simulink library "FPGA_Open_Speech_Tools"  (R2020b)
settings: Solver=VariableStepAuto  StartTime=0.0  StopTime=10.0  RelTol=1e-3
undefined symbols (not defined in the file or in its folder): a, b, c, tableInit
libraries: hdlsllib x159, simulink x26, $bdroot x3
(part 2 of 4)

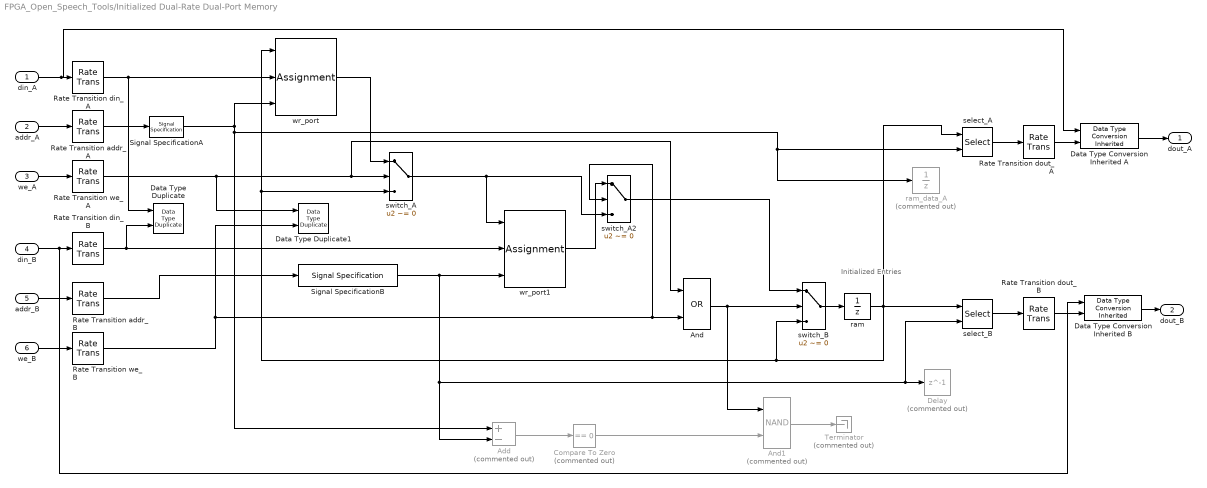
== system FPGA_Open_Speech_Tools/Initialized Dual-Rate Dual-Port Memory ==
  note: Initialized
      | Entries
  din_A : Inport
  addr_A : Inport  Port=2
  we_A : Inport  Port=3  OutDataTypeStr=boolean
  din_B : Inport  Port=4
  addr_B : Inport  Port=5
  we_B : Inport  Port=6  OutDataTypeStr=boolean
  Add : Sum  Commented=on  Inputs=+-
  And : Logic  Operator=OR  AllPortsSameDT=off  OutDataTypeStr=boolean
  And1 : Logic  Commented=on  Operator=NAND  AllPortsSameDT=off  OutDataTypeStr=boolean
  Compare To Zero : simulink/Logic and Bit Operations/Compare To Zero  Commented=on  relop===  OutDataTypeStr=boolean
  Data Type Conversion Inherited A : simulink/Signal Attributes/Data Type Conversion Inherited  ConvertRealWorld=Real World Value  DoSatur=off
      settings: SourceProductBaseCode=SL
  Data Type Conversion Inherited B : simulink/Signal Attributes/Data Type Conversion Inherited  ConvertRealWorld=Real World Value  DoSatur=off
      settings: SourceProductBaseCode=SL
  Data Type Duplicate : DataTypeDuplicate
  Data Type Duplicate1 : DataTypeDuplicate
  Delay : Delay  Commented=on  DelayLength=1
  Rate Transition addr_A : RateTransition  Integrity=off
  Rate Transition addr_B : RateTransition  Integrity=off
  Rate Transition din_A : RateTransition  Integrity=off
  Rate Transition din_B : RateTransition  Integrity=off
  Rate Transition dout_A : RateTransition  Integrity=off
  Rate Transition dout_B : RateTransition  Integrity=off
  Rate Transition we_A : RateTransition  Integrity=off
  Rate Transition we_B : RateTransition  Integrity=off
  Signal SpecificationA : SignalSpecification  OutDataTypeStr=fixdt(0,ram_size,0)  Dimensions=1
  Signal SpecificationB : SignalSpecification  OutDataTypeStr=fixdt(0,ram_size,0)  Dimensions=1
  Terminator : Terminator  Commented=on
      mask Display: disp(sprintf(['Programmable Look-Up Table\nMemory Used: %d bits, Address Width: %d\n' tableFnParam ': %.2d <= x <= %.2d\n Maximum Error: %.2d %%'], 2*2^RAM_SIZE*W_bits, RAM_SIZE, minVal, maxVal, 100*maxErr)); port_label('input',1,'Data_In'); port_label('input',2,'Table_Wr_Data'); port_label('input',3,'Table_RW_Addr'); port_label('input',4,'Table_Wr_En'); port_label('output',1,'Data_Out'); port_label('output',2,'Table_RW_Dout');
  ram : UnitDelay  InitialCondition=Table_Init  SampleTime=-1  HasFrameUpgradeWarning=on
  ram_data_A : UnitDelay  Commented=on  SampleTime=-1  HasFrameUpgradeWarning=on
  select_A : Selector  IndexMode=Zero-based  InputPortWidth=2^ram_size  IndexOptions=Index vector (port)  Indices=[1 3]  OutputSizes=1
  select_B : Selector  IndexMode=Zero-based  InputPortWidth=2^ram_size  IndexOptions=Index vector (port)  Indices=[1 3]  OutputSizes=1
  switch_A : Switch  Criteria=u2 ~= 0
  switch_A2 : Switch  Criteria=u2 ~= 0
  switch_B : Switch  Criteria=u2 ~= 0
  wr_port : Assignment  IndexMode=Zero-based  IndexOptions=Index vector (port)  Indices=1  OutputSizes=[1 1]
  wr_port1 : Assignment  IndexMode=Zero-based  IndexOptions=Index vector (port)  Indices=1  OutputSizes=[1 1]
  dout_A : Outport  VectorParamsAs1DForOutWhenUnconnected=off
  dout_B : Outport  Port=2  VectorParamsAs1DForOutWhenUnconnected=off
  wires:
  Data Type Conversion Inherited A/1 -> dout_A/1
  wr_port1/1 -> switch_A2/1
  Rate Transition dout_A/1 -> Data Type Conversion Inherited A/2
  Data Type Conversion Inherited B/1 -> dout_B/1
  select_B/1 -> Rate Transition dout_B/1
  And/1 -> And1/1, switch_B/2
  Rate Transition addr_A/1 -> Signal SpecificationA/1
  Rate Transition we_A/1 -> And/1, switch_A/2, Data Type Duplicate1/1
  din_A/1 -> Data Type Conversion Inherited A/1, Rate Transition din_A/1
  addr_A/1 -> Rate Transition addr_A/1
  Rate Transition din_B/1 -> wr_port1/2, Data Type Duplicate/2
  switch_A/1 -> wr_port1/1, switch_A2/3
  Signal SpecificationB/1 -> Add/2, select_B/2, Delay/1, wr_port1/3
  switch_A2/1 -> switch_B/1
  Rate Transition din_A/1 -> Data Type Duplicate/1, wr_port/2
  addr_B/1 -> Rate Transition addr_B/1
  switch_B/1 -> ram/1
  Rate Transition dout_B/1 -> Data Type Conversion Inherited B/2
  And1/1 -> Terminator/1
  Add/1 -> Compare To Zero/1
  Compare To Zero/1 -> And1/2
  select_A/1 -> Rate Transition dout_A/1
  ram/1 -> select_B/1, switch_B/3, switch_A/3, wr_port/1, select_A/1
  we_B/1 -> Rate Transition we_B/1
  Signal SpecificationA/1 -> select_A/2, ram_data_A/1, Add/1, wr_port/3
  wr_port/1 -> switch_A/1
  Rate Transition we_B/1 -> switch_A2/2, And/2, Data Type Duplicate1/2
  Rate Transition addr_B/1 -> Signal SpecificationB/1
  din_B/1 -> Data Type Conversion Inherited B/1, Rate Transition din_B/1
  we_A/1 -> Rate Transition we_A/1

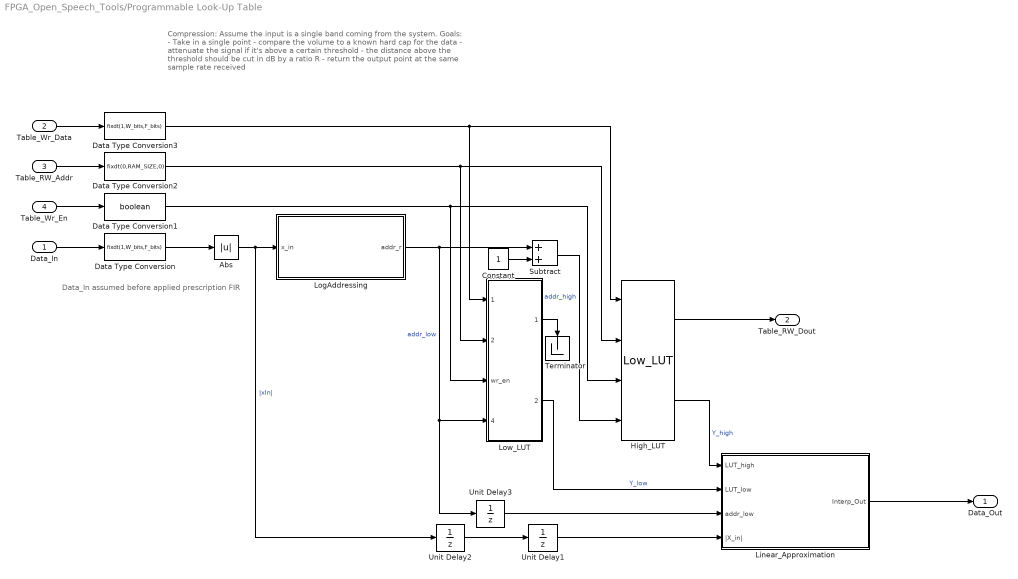
== system FPGA_Open_Speech_Tools/Programmable Look-Up Table ==
  note: Data_In assumed before applied prescription FIR
  note: Compression: Assume the input is a single band coming from the system.
      |
      | Goals:
      | 	- Take in a single point
      | 	- compare the volume to a known hard cap for the data
      | 	- attenuate the signal if it's above a certain threshold
      | 		- the distance above the threshold should be cut in dB by a ratio R
      | 	- return the output point at the same sample rate received
  Data_In : Inport
  Table_Wr_Data : Inport  Port=2
  Table_RW_Addr : Inport  Port=3
  Table_Wr_En : Inport  Port=4
  Abs : Abs
  Constant : Constant  OutDataTypeStr=fixdt(0,RAM_SIZE,0)  SampleTime=-1
  Data Type Conversion : DataTypeConversion  OutDataTypeStr=fixdt(1,W_bits,F_bits)
  Data Type Conversion1 : DataTypeConversion  OutDataTypeStr=boolean
  Data Type Conversion2 : DataTypeConversion  OutDataTypeStr=fixdt(0,RAM_SIZE,0)
  Data Type Conversion3 : DataTypeConversion  OutDataTypeStr=fixdt(1,W_bits,F_bits)
  High_LUT : $bdroot/Programmable Look-Up Table/Low_LUT  ram_size=RAM_SIZE  Table_Init=tableInit
  Linear_Approximation : Subsystem
  LogAddressing : Subsystem
  Low_LUT : Subsystem  mask(Dual-port RAM){ram_size=RAM_SIZE, Table_Init=tableInit}
      mask prompts: ram_size "Address port width (2 to 29 bits)"; Table_Init "Table Initialized Values"
      mask help: This block simulates a dual-port RAM with two data output ports.
      mask init:
      | hdlblkmask_dpram;
      mask Help: helpview([docroot '/simulink/helptargets.map'],'HDL_dual_port_RAM');
  Subtract : Sum  OutDataTypeStr=Inherit: Same as first input
  Terminator : Terminator
  Unit Delay1 : UnitDelay  InitialCondition=1  SampleTime=-1  HasFrameUpgradeWarning=on
  Unit Delay2 : UnitDelay  InitialCondition=1  SampleTime=-1  HasFrameUpgradeWarning=on
  Unit Delay3 : UnitDelay  InitialCondition=1  SampleTime=-1  HasFrameUpgradeWarning=on
  Data_Out : Outport  VectorParamsAs1DForOutWhenUnconnected=off
  Table_RW_Dout : Outport  Port=2  VectorParamsAs1DForOutWhenUnconnected=off
  wires:
  Table_Wr_Data/1 -> Data Type Conversion3/1
  Table_Wr_En/1 -> Data Type Conversion1/1
  Table_RW_Addr/1 -> Data Type Conversion2/1
  LogAddressing/1(addr_r) -> Unit Delay3/1, Low_LUT/4(rd_addr), Subtract/1  "addr_low"
  Abs/1 -> Unit Delay2/1, LogAddressing/1(x_in)  "|xIn|"
  Data_In/1 -> Data Type Conversion/1
  Constant/1 -> Subtract/2
  Subtract/1 -> High_LUT/4  "addr_high"
  Low_LUT/1(wr_dout) -> Terminator/1
  High_LUT/1 -> Table_RW_Dout/1
  High_LUT/2 -> Linear_Approximation/1(LUT_high)  "Y_high"
  Low_LUT/2(rd_dout) -> Linear_Approximation/2(LUT_low)  "Y_low"
  Linear_Approximation/1(Interp_Out) -> Data_Out/1
  Unit Delay2/1 -> Unit Delay1/1
  Unit Delay1/1 -> Linear_Approximation/4(|X_in|)
  Unit Delay3/1 -> Linear_Approximation/3(addr_low)
  Data Type Conversion/1 -> Abs/1
  Data Type Conversion1/1 -> High_LUT/3, Low_LUT/3(wr_en)
  Data Type Conversion2/1 -> High_LUT/2, Low_LUT/2(wr_addr)
  Data Type Conversion3/1 -> High_LUT/1, Low_LUT/1(wr_din)

== system FPGA_Open_Speech_Tools/Programmable Look-Up Table, Linear Scale ==
  note: Data_In assumed before applied prescription FIR
  note: Compression: Assume the input is a single band coming from the system.
      |
      | Goals:
      | 	- Take in a single point
      | 	- compare the volume to a known hard cap for the data
      | 	- attenuate the signal if it's above a certain threshold
      | 		- the distance above the threshold should be cut in dB by a ratio R
      | 	- return the output point at the same sample rate received
  Data_In : Inport
  Table_Wr_Data : Inport  Port=2
  Table_Wr_Addr : Inport  Port=3
  Table_Wr_En : Inport  Port=4
  Data Type Conversion : DataTypeConversion  OutDataTypeStr=fixdt(isSigned,W_bits,F_bits)
  Data Type Conversion1 : DataTypeConversion  OutDataTypeStr=boolean
  Data Type Conversion2 : DataTypeConversion  OutDataTypeStr=fixdt(0,RAM_SIZE,0)
  Data Type Conversion3 : DataTypeConversion  OutDataTypeStr=fixdt(1,W_bits,F_bits)
  LinAddressing : Subsystem
  Low_LUT : Subsystem  mask(Dual-port RAM){ram_size=RAM_SIZE, Table_Init=tableInit}
      mask prompts: ram_size "Address port width (2 to 29 bits)"; Table_Init "Table Initialized Values"
      mask help: This block simulates a dual-port RAM with two data output ports.
      mask init:
      | hdlblkmask_dpram;
      mask Help: helpview([docroot '/simulink/helptargets.map'],'HDL_dual_port_RAM');
  Data_Out : Outport  VectorParamsAs1DForOutWhenUnconnected=off
  Table_RW_Dout : Outport  Port=2  VectorParamsAs1DForOutWhenUnconnected=off
  wires:
  Table_Wr_Data/1 -> Data Type Conversion3/1
  Table_Wr_En/1 -> Data Type Conversion1/1
  Table_Wr_Addr/1 -> Data Type Conversion2/1
  LinAddressing/1(addr_r) -> Low_LUT/4(rd_addr)  "addr"
  Data Type Conversion/1 -> LinAddressing/1(x_in)  "x_in"
  Data_In/1 -> Data Type Conversion/1
  Low_LUT/1(wr_dout) -> Table_RW_Dout/1
  Data Type Conversion1/1 -> Low_LUT/3(wr_en)
  Data Type Conversion2/1 -> Low_LUT/2(wr_addr)
  Data Type Conversion3/1 -> Low_LUT/1(wr_din)
  Low_LUT/2(rd_dout) -> Data_Out/1  "Y_low"

== system FPGA_Open_Speech_Tools/Programmable Lookup Table dB ==
  note: Data_In assumed before applied prescription FIR
  note: Compression: Assume the input is a single band coming from the system.
      |
      | Goals:
      | 	- Take in a single point
      | 	- compare the volume to a known hard cap for the data
      | 	- attenuate the signal if it's above a certain threshold
      | 		- the distance above the threshold should be cut in dB by a ratio R
      | 	- return the output point at the same sample rate received
  Data_In : Inport
  Table_Wr_Data : Inport  Port=2
  Table_RW_Addr : Inport  Port=3
  Table_Wr_En : Inport  Port=4
  Abs : Abs
  Constant : Constant  OutDataTypeStr=fixdt(0,RAM_SIZE,0)  SampleTime=-1
  Data Type Conversion : DataTypeConversion  OutDataTypeStr=fixdt(1,W_bits,F_bits)
  Data Type Conversion1 : DataTypeConversion  OutDataTypeStr=boolean
  Data Type Conversion2 : DataTypeConversion  OutDataTypeStr=fixdt(0,RAM_SIZE,0)
  Data Type Conversion3 : DataTypeConversion  OutDataTypeStr=fixdt(1,W_bits,F_bits-5)
  High_LUT : $bdroot/Programmable Look-Up Table/Low_LUT  ram_size=RAM_SIZE  Table_Init=tableInit
  Linear_Approximation : Subsystem  AncestorBlock=FPGA_Open_Speech_Tools/Programmable Look-Up Table/Linear_Approximation
  LogAddressing : Subsystem  AncestorBlock=FPGA_Open_Speech_Tools/Programmable Look-Up Table/LogAddressing
  Low_LUT : $bdroot/Programmable Look-Up Table/Low_LUT  ram_size=RAM_SIZE  Table_Init=tableInit
  Subtract : Sum  OutDataTypeStr=Inherit: Same as first input
  Terminator : Terminator
  Unit Delay1 : UnitDelay  InitialCondition=1  SampleTime=-1  HasFrameUpgradeWarning=on
  Unit Delay2 : UnitDelay  InitialCondition=1  SampleTime=-1  HasFrameUpgradeWarning=on
  Unit Delay3 : UnitDelay  InitialCondition=1  SampleTime=-1  HasFrameUpgradeWarning=on
  Data_Out : Outport  VectorParamsAs1DForOutWhenUnconnected=off
  Table_RW_Dout : Outport  Port=2  VectorParamsAs1DForOutWhenUnconnected=off
  wires:
  Data Type Conversion1/1 -> High_LUT/3, Low_LUT/3
  Table_RW_Addr/1 -> Data Type Conversion2/1
  Data Type Conversion3/1 -> High_LUT/1, Low_LUT/1
  Constant/1 -> Subtract/2
  Table_Wr_En/1 -> Data Type Conversion1/1
  High_LUT/2 -> Linear_Approximation/1(LUT_high)  "Y_high"
  LogAddressing/1(addr_r) -> Unit Delay3/1, Low_LUT/4, Subtract/1  "addr_low"
  High_LUT/1 -> Table_RW_Dout/1
  Subtract/1 -> High_LUT/4  "addr_high"
  Data Type Conversion/1 -> Abs/1
  Unit Delay1/1 -> Linear_Approximation/4(|X_in|)
  Low_LUT/1 -> Terminator/1
  Low_LUT/2 -> Linear_Approximation/2(LUT_low)  "Y_low"
  Unit Delay3/1 -> Linear_Approximation/3(addr_low)
  Abs/1 -> Unit Delay2/1, LogAddressing/1(x_in)  "|xIn|"
  Data Type Conversion2/1 -> High_LUT/2, Low_LUT/2
  Linear_Approximation/1(Interp_Out) -> Data_Out/1
  Unit Delay2/1 -> Unit Delay1/1
  Data_In/1 -> Data Type Conversion/1
  Table_Wr_Data/1 -> Data Type Conversion3/1

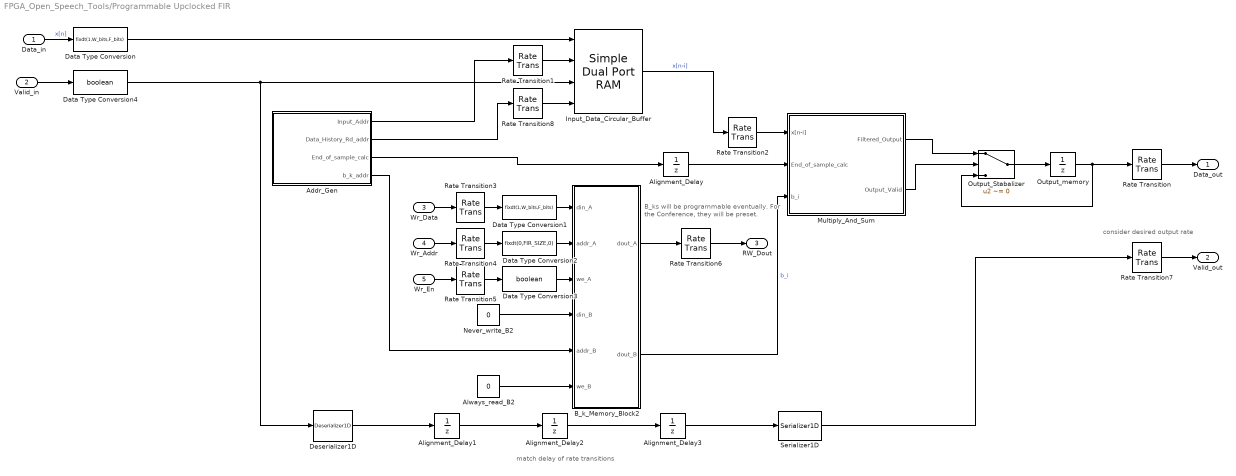
== system FPGA_Open_Speech_Tools/Programmable Upclocked FIR ==
  note: match delay of rate transitions
  note: consider desired output rate
  note: B_ks will be programmable eventually.
      | For the Conference, they will be preset.
  Data_in : Inport
  Valid_in : Inport  Port=2
  Wr_Data : Inport  Port=3
  Wr_Addr : Inport  Port=4
  Wr_En : Inport  Port=5
  "Addr_Gen " : Subsystem
  Alignment_Delay{,1..3} (4 alike) : UnitDelay  SampleTime=-1  HasFrameUpgradeWarning=on
  Always_read_B2 : Constant  Value=0  OutDataTypeStr=boolean  SampleTime=Ts/FIR_UPRATE
  B_k_Memory_Block2 : Subsystem  mask(Dual-rate dual-port RAM){ram_size=FIR_SIZE, B_k_init=firCoeff}
      mask prompts: ram_size "Address port width (2 to 28 bits)"
      mask help: This block simulates a dual-clock dual-port RAM with two data output ports.
      mask init:
      | hdlblkmask_drdpram();
      mask Help: helpview([docroot '/simulink/helptargets.map'],'HDL_dual_rate_dual_port_ram');
  Data Type Conversion : DataTypeConversion  OutDataTypeStr=fixdt(1,W_bits,F_bits)
  Data Type Conversion1 : DataTypeConversion  OutDataTypeStr=fixdt(1,W_bits,F_bits)
  Data Type Conversion2 : DataTypeConversion  OutDataTypeStr=fixdt(0,FIR_SIZE,0)
  Data Type Conversion3 : DataTypeConversion  OutDataTypeStr=boolean
  Data Type Conversion4 : DataTypeConversion  OutDataTypeStr=boolean
  Deserializer1D : hdlsllib/HDL Operations/Deserializer1D  Ratio=(1/maxRate)/Ts_system  IdleCycles=0  InitialCondition=0  startIn=off  validIn=off  validOut=off  inputDataDimensions=-1  inputSampleTime=-1  inputSignalType=auto
      settings: SourceProductBaseCode=SL
  Input_Data_Circular_Buffer : hdlsllib/HDL RAMs/Simple Dual Port RAM  ram_size=FIR_SIZE
      settings: SourceProductBaseCode=SL
  Multiply_And_Sum : Subsystem
  Never_write_B2 : Constant  Value=0  OutDataTypeStr=fixdt(1, W_bits, F_bits)  SampleTime=Ts/FIR_UPRATE
  Output_Stabalizer : Switch  Criteria=u2 ~= 0
  Output_memory : UnitDelay  SampleTime=-1  HasFrameUpgradeWarning=on
  Rate Transition{,1,6..8} (5 alike) : RateTransition  OutPortSampleTime=Ts_system
  Rate Transition{2..5} (4 alike) : RateTransition  OutPortSampleTime=Ts/FIR_UPRATE
  Serializer1D : hdlsllib/HDL Operations/Serializer1D  Ratio=(1/maxRate)/Ts_system  IdleCycles=0  validIn=off  startOut=off  validOut=off  inputDataDimensions=-1  inputSampleTime=-1  inputSignalType=auto
      settings: SourceProductBaseCode=SL
  Data_out : Outport  VectorParamsAs1DForOutWhenUnconnected=off
  Valid_out : Outport  Port=2  VectorParamsAs1DForOutWhenUnconnected=off
  RW_Dout : Outport  Port=3  VectorParamsAs1DForOutWhenUnconnected=off
  wires:
  Alignment_Delay/1 -> Multiply_And_Sum/2(End_of_sample_calc)
  "Addr_Gen "/4(b_k_addr) -> B_k_Memory_Block2/5(addr_B)
  Output_memory/1 -> Rate Transition/1, Output_Stabalizer/3
  Valid_in/1 -> Data Type Conversion4/1
  Never_write_B2/1 -> B_k_Memory_Block2/4(din_B)
  Multiply_And_Sum/1(Filtered_Output) -> Output_Stabalizer/1
  Data_in/1 -> Data Type Conversion/1  "x[n]"
  "Addr_Gen "/3(End_of_sample_calc) -> Alignment_Delay/1
  B_k_Memory_Block2/2(dout_B) -> Multiply_And_Sum/3(b_i)  "b_i"
  "Addr_Gen "/1(Input_Addr) -> Rate Transition1/1
  Output_Stabalizer/1 -> Output_memory/1
  "Addr_Gen "/2(Data_History_Rd_addr) -> Rate Transition8/1
  Rate Transition4/1 -> Data Type Conversion2/1
  Input_Data_Circular_Buffer/1 -> Rate Transition2/1  "x[n-i]"
  Rate Transition3/1 -> Data Type Conversion1/1
  Always_read_B2/1 -> B_k_Memory_Block2/6(we_B)
  Rate Transition/1 -> Data_out/1
  Wr_Data/1 -> Rate Transition3/1
  Wr_Addr/1 -> Rate Transition4/1
  Rate Transition5/1 -> Data Type Conversion3/1
  Wr_En/1 -> Rate Transition5/1
  B_k_Memory_Block2/1(dout_A) -> Rate Transition6/1
  Rate Transition6/1 -> RW_Dout/1
  Rate Transition7/1 -> Valid_out/1
  Data Type Conversion1/1 -> B_k_Memory_Block2/1(din_A)
  Data Type Conversion2/1 -> B_k_Memory_Block2/2(addr_A)
  Data Type Conversion3/1 -> B_k_Memory_Block2/3(we_A)
  Multiply_And_Sum/2(Output_Valid) -> Output_Stabalizer/2
  Data Type Conversion4/1 -> Deserializer1D/1, Input_Data_Circular_Buffer/3
  Data Type Conversion/1 -> Input_Data_Circular_Buffer/1
  Deserializer1D/1 -> Alignment_Delay1/1
  Serializer1D/1 -> Rate Transition7/1
  Rate Transition2/1 -> Multiply_And_Sum/1(x[n-i])
  Rate Transition1/1 -> Input_Data_Circular_Buffer/2
  Rate Transition8/1 -> Input_Data_Circular_Buffer/4
  Alignment_Delay1/1 -> Alignment_Delay2/1
  Alignment_Delay2/1 -> Alignment_Delay3/1
  Alignment_Delay3/1 -> Serializer1D/1

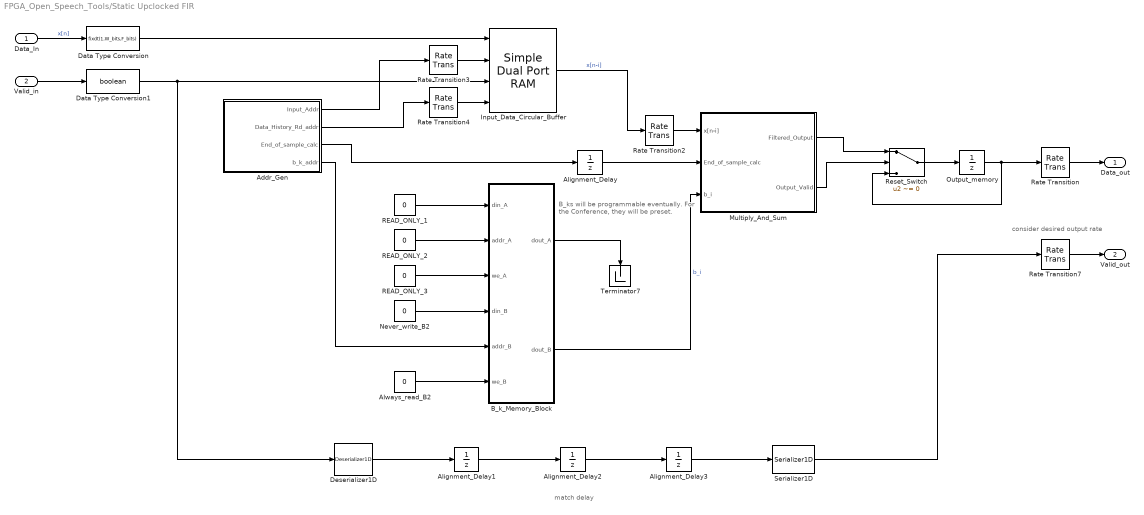
== system FPGA_Open_Speech_Tools/Static Upclocked FIR ==
  note: consider desired output rate
  note: B_ks will be programmable eventually.
      | For the Conference, they will be preset.
  note: match delay
  Data_In : Inport
  Valid_in : Inport  Port=2
  "Addr_Gen " : Subsystem
  Alignment_Delay{,1..3} (4 alike) : UnitDelay  SampleTime=-1  HasFrameUpgradeWarning=on
  Always_read_B2 : Constant  Value=0  OutDataTypeStr=boolean  SampleTime=Ts/FIR_UPRATE
  B_k_Memory_Block : Subsystem  mask(Dual-rate dual-port RAM){ram_size=FIR_SIZE, B_k_init=firCoeff}
      mask prompts: ram_size "Address port width (2 to 28 bits)"
      mask help: This block simulates a dual-clock dual-port RAM with two data output ports.
      mask init:
      | hdlblkmask_drdpram();
      mask Help: helpview([docroot '/simulink/helptargets.map'],'HDL_dual_rate_dual_port_ram');
  Data Type Conversion : DataTypeConversion  OutDataTypeStr=fixdt(1,W_bits,F_bits)
  Data Type Conversion1 : DataTypeConversion  OutDataTypeStr=boolean
  Deserializer1D : hdlsllib/HDL Operations/Deserializer1D  Ratio=(1/maxRate)/Ts_system  IdleCycles=0  InitialCondition=0  startIn=off  validIn=off  validOut=off  inputDataDimensions=-1  inputSampleTime=-1  inputSignalType=auto
      settings: SourceProductBaseCode=SL
  Input_Data_Circular_Buffer : hdlsllib/HDL RAMs/Simple Dual Port RAM  ram_size=FIR_SIZE
      settings: SourceProductBaseCode=SL
  Multiply_And_Sum : Subsystem
  Never_write_B2 : Constant  Value=0  OutDataTypeStr=fixdt(1, W_bits, F_bits)  SampleTime=Ts/FIR_UPRATE
  Output_memory : UnitDelay  SampleTime=-1  HasFrameUpgradeWarning=on
  READ_ONLY_1 : Constant  Value=0  OutDataTypeStr=fixdt(1, W_bits, F_bits)  SampleTime=Ts/FIR_UPRATE
  READ_ONLY_2 : Constant  Value=0  OutDataTypeStr=fixdt(0,FIR_SIZE, 0)  SampleTime=Ts/FIR_UPRATE
  READ_ONLY_3 : Constant  Value=0  OutDataTypeStr=boolean  SampleTime=Ts/FIR_UPRATE
  Rate Transition : RateTransition  OutPortSampleTime=Ts_system
  Rate Transition2 : RateTransition  OutPortSampleTime=Ts/FIR_UPRATE
  Rate Transition3 : RateTransition  OutPortSampleTime=Ts/FIR_UPRATE
  Rate Transition4 : RateTransition  OutPortSampleTime=Ts/FIR_UPRATE
  Rate Transition7 : RateTransition  OutPortSampleTime=Ts_system
  Reset_Switch : Switch  Criteria=u2 ~= 0
  Serializer1D : hdlsllib/HDL Operations/Serializer1D  Ratio=(1/maxRate)/Ts_system  IdleCycles=0  validIn=off  startOut=off  validOut=off  inputDataDimensions=-1  inputSampleTime=-1  inputSignalType=auto
      settings: SourceProductBaseCode=SL
  Terminator7 : Terminator
  Data_out : Outport  VectorParamsAs1DForOutWhenUnconnected=off
  Valid_out : Outport  Port=2  VectorParamsAs1DForOutWhenUnconnected=off
  wires:
  Valid_in/1 -> Data Type Conversion1/1
  Alignment_Delay/1 -> Multiply_And_Sum/2(End_of_sample_calc)
  "Addr_Gen "/4(b_k_addr) -> B_k_Memory_Block/5(addr_B)
  Output_memory/1 -> Rate Transition/1, Reset_Switch/3
  Never_write_B2/1 -> B_k_Memory_Block/4(din_B)
  READ_ONLY_3/1 -> B_k_Memory_Block/3(we_A)
  Multiply_And_Sum/1(Filtered_Output) -> Reset_Switch/1
  Data_In/1 -> Data Type Conversion/1  "x[n]"
  "Addr_Gen "/3(End_of_sample_calc) -> Alignment_Delay/1
  B_k_Memory_Block/2(dout_B) -> Multiply_And_Sum/3(b_i)  "b_i"
  "Addr_Gen "/1(Input_Addr) -> Rate Transition3/1
  Reset_Switch/1 -> Output_memory/1
  "Addr_Gen "/2(Data_History_Rd_addr) -> Rate Transition4/1
  READ_ONLY_2/1 -> B_k_Memory_Block/2(addr_A)
  Input_Data_Circular_Buffer/1 -> Rate Transition2/1  "x[n-i]"
  READ_ONLY_1/1 -> B_k_Memory_Block/1(din_A)
  Multiply_And_Sum/2(Output_Valid) -> Reset_Switch/2
  B_k_Memory_Block/1(dout_A) -> Terminator7/1
  Always_read_B2/1 -> B_k_Memory_Block/6(we_B)
  Rate Transition/1 -> Data_out/1
  Rate Transition7/1 -> Valid_out/1
  Data Type Conversion/1 -> Input_Data_Circular_Buffer/1
  Data Type Conversion1/1 -> Deserializer1D/1, Input_Data_Circular_Buffer/3
  Rate Transition3/1 -> Input_Data_Circular_Buffer/2
  Rate Transition4/1 -> Input_Data_Circular_Buffer/4
  Rate Transition2/1 -> Multiply_And_Sum/1(x[n-i])
  Alignment_Delay2/1 -> Alignment_Delay3/1
  Alignment_Delay3/1 -> Serializer1D/1
  Alignment_Delay1/1 -> Alignment_Delay2/1
  Deserializer1D/1 -> Alignment_Delay1/1
  Serializer1D/1 -> Rate Transition7/1

== system FPGA_Open_Speech_Tools/Variable Delay Block ==
  note: Special Case for Delay = 2^N:
      | If Valid is asserted, we have 1 clock cycle before overwriting the circ buffer data for 2^N samples ago.
      | Readout of circ buffer will be correct for 1 cycle.
      |
      | If valid is not asserted?
      | This means the data for 2^N samples ago has already been overwritten. It's already too late to get that sample.
  note: Solution: Implement Special Case switches to allow for read-first enabled circular buffer 1 cycle to write.
      | Then, use a switch to allow the circ buffer to take back over, preventing non-valid signals from showing on output.
  note: max delay: (2^N) -1
  note: circ buffer is read-first, requiring a switch for delays of 0 and 1
  note: problem: no delay of 1 available with circular buffer
  Data_In : Inport
  Data_Valid : Inport  Port=2
  Delay : Inport  Port=3
  "Addr_Gen " : Subsystem
  Data Type Conversion : DataTypeConversion  OutDataTypeStr=fixdt(0, RAM_SIZE, 0)
  Data Type Conversion1 : DataTypeConversion  OutDataTypeStr=boolean
  Input_Data_Circular_Buffer : Subsystem
  Multiport Switch : MultiPortSwitch  DataPortOrder=Zero-based contiguous  Inputs=2  DataPortIndices={0,2^RAMSIZE}  DiagnosticForDefault=None  zeroidx=on
  Output_Stabalizer_Z0 : Switch  Criteria=u2 ~= 0
  Subtract : Sum  Inputs=+-  OutDataTypeStr=Inherit: Same as first input
  Data_out : Outport  VectorParamsAs1DForOutWhenUnconnected=off
  wires:
  Subtract/1 -> Input_Data_Circular_Buffer/4(rd_addr)
  Data_Valid/1 -> Data Type Conversion1/1
  Input_Data_Circular_Buffer/1(rd_dout) -> Multiport Switch/3, Output_Stabalizer_Z0/3  "x[n-i]"
  Delay/1 -> Data Type Conversion/1
  Multiport Switch/1 -> Data_out/1
  Data Type Conversion/1 -> Multiport Switch/1, Subtract/2
  Data_In/1 -> Input_Data_Circular_Buffer/1(wr_din), Output_Stabalizer_Z0/1
  Data Type Conversion1/1 -> Input_Data_Circular_Buffer/3(wr_en), Output_Stabalizer_Z0/2, "Addr_Gen "/Enable
  Output_Stabalizer_Z0/1 -> Multiport Switch/2
  "Addr_Gen "/1(Input_Addr) -> Subtract/1, Input_Data_Circular_Buffer/2(wr_addr)

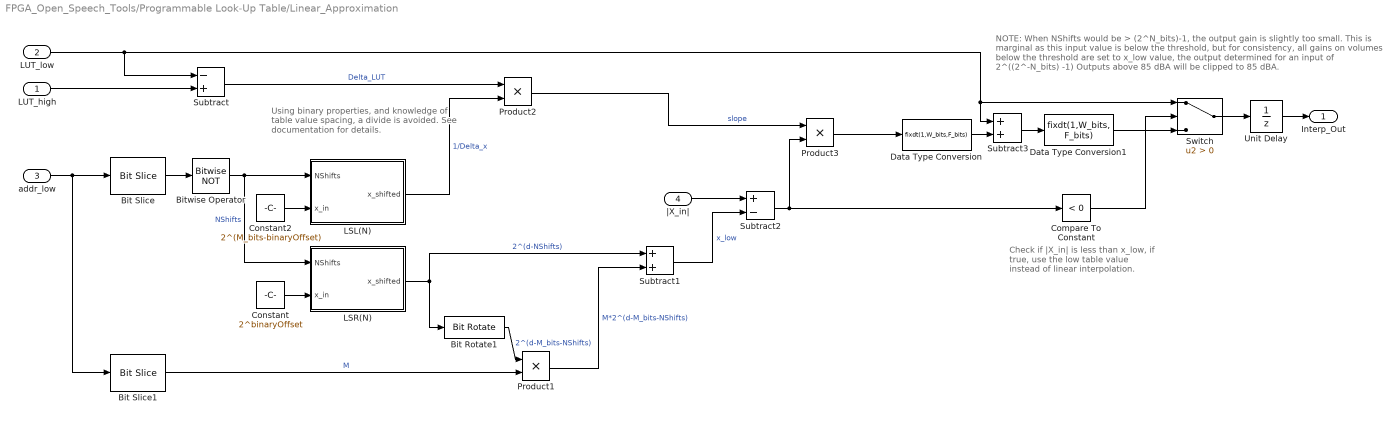
== system FPGA_Open_Speech_Tools/Programmable Look-Up Table/Linear_Approximation ==
  note: Using binary properties, and knowledge
      | of table value spacing, a divide is avoided.
      | See documentation for details.
  note: Check if |X_in| is less than x_low,
      | if true, use the low table value
      | instead of linear interpolation.
  note: NOTE: When NShifts would be > (2^N_bits)-1, the output gain is slightly too small.
      | This is marginal as this input value is below the threshold, but for consistency,
      | all gains on volumes below the threshold are set to x_low value, the output determined
      | for an input of 2^((2^-N_bits)  -1)
      | Outputs above 85 dBA will be clipped to 85 dBA.
  LUT_high : Inport
  LUT_low : Inport  Port=2
  addr_low : Inport  Port=3
  |X_in| : Inport  Port=4
  Bit Rotate1 : hdlsllib/Logic and Bit Operations/Bit Rotate  mode=Rotate Right  N=M_bits
      settings: SourceProductBaseCode=SL
  Bit Slice : hdlsllib/Logic and Bit Operations/Bit Slice  lidx=M_bits+N_bits-1  ridx=M_bits
      settings: SourceProductBaseCode=SL
  Bit Slice1 : hdlsllib/Logic and Bit Operations/Bit Slice  lidx=M_bits-1  ridx=0
      settings: SourceProductBaseCode=SL
  Bitwise Operator : simulink/Logic and Bit Operations/Bitwise Operator  logicop=NOT  UseBitMask=off  BitMask=bin2dec('11011001')  BitMaskRealWorld=Stored Integer
  Compare To Constant : simulink/Logic and Bit Operations/Compare To Constant  relop=<  const=0  OutDataTypeStr=boolean
  Constant : Constant  Value=2^binaryOffset  OutDataTypeStr=fixdt(0,W_bits,W_bits-2)  SampleTime=-1
  Constant2 : Constant  Value=2^(M_bits-binaryOffset)  OutDataTypeStr=fixdt(0,W_bits,0)  SampleTime=-1
  Data Type Conversion : DataTypeConversion  OutDataTypeStr=fixdt(1,W_bits,F_bits)
  Data Type Conversion1 : DataTypeConversion  OutDataTypeStr=fixdt(1,W_bits, F_bits)
  LSL(N) : Subsystem
  LSR(N) : Subsystem
  Product1 : Product
  Product2 : Product
  Product3 : Product
  Subtract : Sum  Inputs=-+  OutDataTypeStr=Inherit: Same as first input
  Subtract1 : Sum  OutDataTypeStr=fixdt(1,W_bits, F_bits)
  Subtract2 : Sum  Inputs=+-  OutDataTypeStr=Inherit: Same as first input
  Subtract3 : Sum
  Switch : Switch  Criteria=u2 > Threshold
  Unit Delay : UnitDelay  InitialCondition=1  SampleTime=-1  HasFrameUpgradeWarning=on
  Interp_Out : Outport  VectorParamsAs1DForOutWhenUnconnected=off
  wires:
  addr_low/1 -> Bit Slice1/1, Bit Slice/1
  Bit Slice/1 -> Bitwise Operator/1
  Bitwise Operator/1 -> LSR(N)/1(NShifts), LSL(N)/1(NShifts)  "NShifts"
  Bit Slice1/1 -> Product1/2  "M"
  LUT_high/1 -> Subtract/2
  LUT_low/1 -> Subtract/1, Switch/1, Subtract3/1
  Subtract/1 -> Product2/1  "Delta_LUT"
  Constant/1 -> LSR(N)/2(x_in)
  LSR(N)/1(x_shifted) -> Subtract1/1, Bit Rotate1/1  "2^(d-NShifts)"
  Bit Rotate1/1 -> Product1/1  "2^(d-M_bits-NShifts)"
  Product1/1 -> Subtract1/2  "M*2^(d-M_bits-NShifts)"
  Subtract1/1 -> Subtract2/2  "x_low"
  LSL(N)/1(x_shifted) -> Product2/2  "1/Delta_x"
  Product2/1 -> Product3/1  "slope"
  |X_in|/1 -> Subtract2/1
  Subtract2/1 -> Compare To Constant/1, Product3/2
  Product3/1 -> Data Type Conversion/1
  Subtract3/1 -> Data Type Conversion1/1
  Constant2/1 -> LSL(N)/2(x_in)
  Data Type Conversion/1 -> Subtract3/2
  Data Type Conversion1/1 -> Switch/3
  Unit Delay/1 -> Interp_Out/1
  Compare To Constant/1 -> Switch/2
  Switch/1 -> Unit Delay/1

== system FPGA_Open_Speech_Tools/Programmable Look-Up Table/LogAddressing ==
  note: z-1 here
      |    	|
      |    	|
      |   	v
  note: If input > highest expected input,
  note: If input < floor threshold input,
      | use the output corresponding to
      | the floor threshold input.
  note: Note: simulation version of this block has no latency.
      | But, in VHDL the inputs are registered, delaying the signal by 1.
      | If testing a simulation, simply attach a unit delay block after the
      | addition and before the signal split.
  note: Have to change size to 40 because
      |  LZC made for 40 bit number
  note: EFFECTIVELY shift_left(x_in,NShifts)
  x_in : Inport
  Bit Concat : hdlsllib/Logic and Bit Operations/Bit Concat  numInputs=2
  Bit Slice : hdlsllib/Logic and Bit Operations/Bit Slice  lidx=N_bits-1  ridx=0
      settings: SourceProductBaseCode=SL
  Bit Slice1 : hdlsllib/Logic and Bit Operations/Bit Slice  lidx=F_bits-1+binaryOffset  ridx=F_bits-M_bits+binaryOffset
      settings: SourceProductBaseCode=SL
  Bitwise Operator1 : simulink/Logic and Bit Operations/Bitwise Operator  logicop=NOT  UseBitMask=off  BitMask=bin2dec('11011001')  BitMaskRealWorld=Stored Integer
  Constant6 : Constant  Value=0  OutDataTypeStr=fixdt(0,RAM_SIZE,0)  SampleTime=-1
  Data Type Conversion : DataTypeConversion  OutDataTypeStr=fixdt(0,40,F_bits+40-W_bits)
  Delay1 : Delay  DelayLength=1  InitialCondition=minVal
  Delay2 : Delay  DelayLength=1  InitialCondition=minVal
  LSL(N) : Subsystem
  MATLAB Function : MATLAB Function  TreatAsAtomicUnit=on
  Offset : Constant  Value=W_bits-1-F_bits-binaryOffset  OutDataTypeStr=fixdt(0,6,0)  SampleTime=-1
  Remove Sign : DataTypeConversion  OutDataTypeStr=fixdt(0,W_bits,F_bits)
  Subtract : Sum  Inputs=+-  OutDataTypeStr=Inherit: Same as first input
  Switch1 : Switch  Criteria=u2 ~= 0
  Threshold Check : simulink/Logic and Bit Operations/Compare To Constant  relop=>  const=2^N_bits -1  OutDataTypeStr=boolean
  addr_r : Outport  VectorParamsAs1DForOutWhenUnconnected=off
  wires:
  x_in/1 -> Remove Sign/1, Data Type Conversion/1
  Bit Slice1/1 -> Bit Concat/2  "M"
  Bitwise Operator1/1 -> Bit Concat/1  "addr(5 downto 2)"
  MATLAB Function/1(lzc_count) -> Subtract/1
  Bit Concat/1 -> Switch1/3
  Offset/1 -> Subtract/2
  Bit Slice/1 -> Bitwise Operator1/1, LSL(N)/1(NShifts)  "NShifts"
  Delay2/1 -> LSL(N)/2(x_in)
  LSL(N)/1(x_shifted) -> Bit Slice1/1
  Data Type Conversion/1 -> MATLAB Function/1(x)
  Constant6/1 -> Switch1/1
  Switch1/1 -> addr_r/1
  Threshold Check/1 -> Switch1/2
  Remove Sign/1 -> Delay2/1
  Subtract/1 -> Delay1/1
  Delay1/1 -> Bit Slice/1, Threshold Check/1

== system FPGA_Open_Speech_Tools/Programmable Look-Up Table/Low_LUT ==
  note: Initialized
  wr_din : Inport
  wr_addr : Inport  Port=2
  wr_en : Inport  Port=3  OutDataTypeStr=boolean
  rd_addr : Inport  Port=4
  Signal Specification : SignalSpecification  OutDataTypeStr=fixdt(0,RAM_SIZE,0)  Dimensions=1
  Signal Specification1 : SignalSpecification  OutDataTypeStr=fixdt(0,RAM_SIZE,0)  Dimensions=1
  convert : DataTypeConversion  OutDataTypeStr=uint16
  convert1 : DataTypeConversion  OutDataTypeStr=uint16
  ram : UnitDelay  InitialCondition=Table_Init  SampleTime=-1  HasFrameUpgradeWarning=on
  ram_data : UnitDelay  SampleTime=-1  HasFrameUpgradeWarning=on
  select : Selector  IndexMode=Zero-based  InputPortWidth=2^ram_size  IndexOptions=Index vector (port)  Indices=[1 3]  OutputSizes=1
  select1 : Selector  IndexMode=Zero-based  InputPortWidth=2^ram_size  IndexOptions=Index vector (port)  Indices=[1 3]  OutputSizes=1
  switch : Switch  Criteria=u2 ~= 0
  wr_addr_d : UnitDelay  SampleTime=-1  HasFrameUpgradeWarning=on
  wr_port : Assignment  IndexMode=Zero-based  IndexOptions=Index vector (port)  Indices=1  OutputSizes=[1 1]
  wr_dout : Outport  VectorParamsAs1DForOutWhenUnconnected=off
  rd_dout : Outport  Port=2  VectorParamsAs1DForOutWhenUnconnected=off
  wires:
  ram_data/1 -> rd_dout/1
  Signal Specification/1 -> convert/1
  wr_addr/1 -> Signal Specification/1
  wr_port/1 -> switch/1
  switch/1 -> ram/1
  ram/1 -> wr_port/1, select/1, select1/1, switch/3
  wr_din/1 -> wr_port/2
  wr_en/1 -> switch/2
  rd_addr/1 -> Signal Specification1/1
  select/1 -> ram_data/1
  convert/1 -> wr_port/3, wr_addr_d/1
  convert1/1 -> select/2
  select1/1 -> wr_dout/1
  wr_addr_d/1 -> select1/2
  Signal Specification1/1 -> convert1/1

== system FPGA_Open_Speech_Tools/Programmable Look-Up Table, Linear Scale/LinAddressing ==
  x_in : Inport
  Bit Slice1 : hdlsllib/Logic and Bit Operations/Bit Slice  lidx=W_bits-1  ridx=W_bits-N_bits
      settings: SourceProductBaseCode=SL
  addr_r : Outport  VectorParamsAs1DForOutWhenUnconnected=off
  wires:
  x_in/1 -> Bit Slice1/1
  Bit Slice1/1 -> addr_r/1

== system FPGA_Open_Speech_Tools/Programmable Look-Up Table, Linear Scale/Low_LUT ==
  note: Initialized
  wr_din : Inport
  wr_addr : Inport  Port=2
  wr_en : Inport  Port=3  OutDataTypeStr=boolean
  rd_addr : Inport  Port=4
  Signal Specification : SignalSpecification  OutDataTypeStr=fixdt(0,ram_size,0)  Dimensions=1
  Signal Specification1 : SignalSpecification  OutDataTypeStr=fixdt(0,ram_size,0)  Dimensions=1
  convert : DataTypeConversion  OutDataTypeStr=uint16
  convert1 : DataTypeConversion  OutDataTypeStr=uint16
  ram : UnitDelay  InitialCondition=Table_Init  SampleTime=-1  HasFrameUpgradeWarning=on
  ram_data : UnitDelay  SampleTime=-1  HasFrameUpgradeWarning=on
  select : Selector  IndexMode=Zero-based  InputPortWidth=2^ram_size  IndexOptions=Index vector (port)  Indices=[1 3]  OutputSizes=1
  select1 : Selector  IndexMode=Zero-based  InputPortWidth=2^ram_size  IndexOptions=Index vector (port)  Indices=[1 3]  OutputSizes=1
  switch : Switch  Criteria=u2 ~= 0
  wr_addr_d : UnitDelay  SampleTime=-1  HasFrameUpgradeWarning=on
  wr_port : Assignment  IndexMode=Zero-based  IndexOptions=Index vector (port)  Indices=1  OutputSizes=[1 1]
  wr_dout : Outport  VectorParamsAs1DForOutWhenUnconnected=off
  rd_dout : Outport  Port=2  VectorParamsAs1DForOutWhenUnconnected=off
  wires:
  ram_data/1 -> rd_dout/1
  Signal Specification/1 -> convert/1
  wr_addr/1 -> Signal Specification/1
  wr_port/1 -> switch/1
  switch/1 -> ram/1
  ram/1 -> wr_port/1, select/1, select1/1, switch/3
  wr_din/1 -> wr_port/2
  wr_en/1 -> switch/2
  rd_addr/1 -> Signal Specification1/1
  select/1 -> ram_data/1
  convert/1 -> wr_port/3, wr_addr_d/1
  convert1/1 -> select/2
  select1/1 -> wr_dout/1
  wr_addr_d/1 -> select1/2
  Signal Specification1/1 -> convert1/1

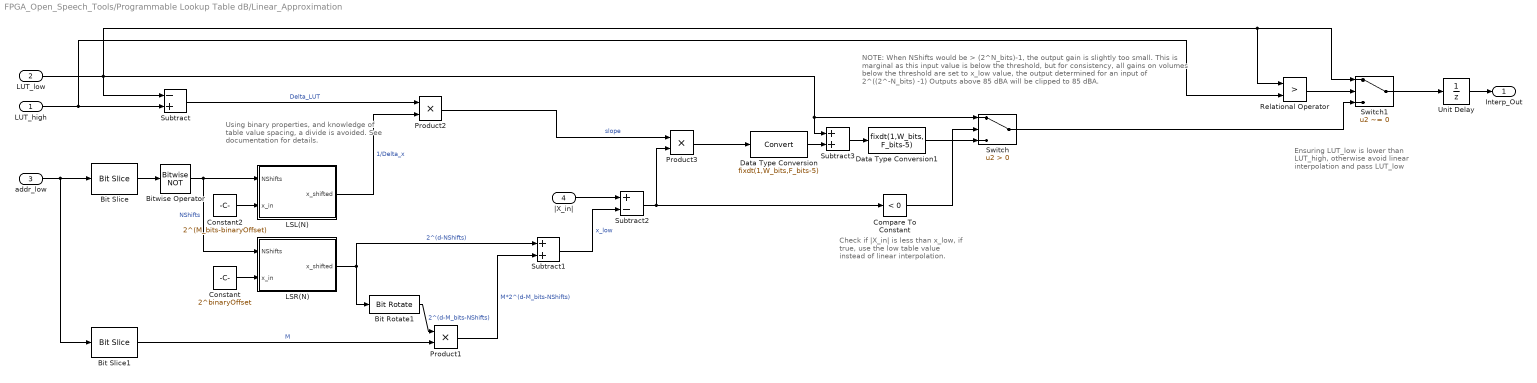
== system FPGA_Open_Speech_Tools/Programmable Lookup Table dB/Linear_Approximation ==
  note: Ensuring LUT_low is lower than
      | LUT_high, otherwise avoid linear
      | interpolation and pass LUT_low
  note: NOTE: When NShifts would be > (2^N_bits)-1, the output gain is slightly too small.
      | This is marginal as this input value is below the threshold, but for consistency,
      | all gains on volumes below the threshold are set to x_low value, the output determined
      | for an input of 2^((2^-N_bits)  -1)
      | Outputs above 85 dBA will be clipped to 85 dBA.
  note: Check if |X_in| is less than x_low,
      | if true, use the low table value
      | instead of linear interpolation.
  note: Using binary properties, and knowledge
      | of table value spacing, a divide is avoided.
      | See documentation for details.
  LUT_high : Inport
  LUT_low : Inport  Port=2
  addr_low : Inport  Port=3
  |X_in| : Inport  Port=4
  Bit Rotate1 : hdlsllib/Logic and Bit Operations/Bit Rotate  mode=Rotate Right  N=M_bits
      settings: SourceProductBaseCode=SL
  Bit Slice : hdlsllib/Logic and Bit Operations/Bit Slice  lidx=M_bits+N_bits-1  ridx=M_bits
      settings: SourceProductBaseCode=SL
  Bit Slice1 : hdlsllib/Logic and Bit Operations/Bit Slice  lidx=M_bits-1  ridx=0
      settings: SourceProductBaseCode=SL
  Bitwise Operator : simulink/Logic and Bit Operations/Bitwise Operator  logicop=NOT  UseBitMask=off  BitMask=bin2dec('11011001')  BitMaskRealWorld=Stored Integer
  Compare To Constant : simulink/Logic and Bit Operations/Compare To Constant  relop=<  const=0  OutDataTypeStr=boolean
  Constant : Constant  Value=2^binaryOffset  OutDataTypeStr=fixdt(0,W_bits,W_bits-3)  SampleTime=-1
  Constant2 : Constant  Value=2^(M_bits-binaryOffset)  OutDataTypeStr=fixdt(0,W_bits,0)  SampleTime=-1
  Data Type Conversion : DataTypeConversion  OutDataTypeStr=fixdt(1,W_bits,F_bits-5)
  Data Type Conversion1 : DataTypeConversion  OutDataTypeStr=fixdt(1,W_bits, F_bits-5)
  LSL(N) : Subsystem
  LSR(N) : Subsystem
  Product1 : Product
  Product2 : Product
  Product3 : Product
  Relational Operator : RelationalOperator  Operator=>  OutDataTypeStr=boolean  RndMeth=Nearest
  Subtract : Sum  Inputs=-+  OutDataTypeStr=Inherit: Same as first input
  Subtract1 : Sum  OutDataTypeStr=fixdt(1,W_bits, F_bits)
  Subtract2 : Sum  Inputs=+-  OutDataTypeStr=Inherit: Same as first input
  Subtract3 : Sum
  Switch : Switch  Criteria=u2 > Threshold
  Switch1 : Switch  Criteria=u2 ~= 0
  Unit Delay : UnitDelay  InitialCondition=1  SampleTime=-1  HasFrameUpgradeWarning=on
  Interp_Out : Outport  VectorParamsAs1DForOutWhenUnconnected=off
  wires:
  Switch/1 -> Switch1/3
  Compare To Constant/1 -> Switch/2
  Unit Delay/1 -> Interp_Out/1
  Data Type Conversion1/1 -> Switch/3
  Data Type Conversion/1 -> Subtract3/2
  Constant2/1 -> LSL(N)/2(x_in)
  Subtract3/1 -> Data Type Conversion1/1
  Product3/1 -> Data Type Conversion/1
  Subtract2/1 -> Product3/2, Compare To Constant/1
  |X_in|/1 -> Subtract2/1
  Product2/1 -> Product3/1  "slope"
  LSL(N)/1(x_shifted) -> Product2/2  "1/Delta_x"
  Subtract1/1 -> Subtract2/2  "x_low"
  Product1/1 -> Subtract1/2  "M*2^(d-M_bits-NShifts)"
  Bit Rotate1/1 -> Product1/1  "2^(d-M_bits-NShifts)"
  LSR(N)/1(x_shifted) -> Bit Rotate1/1, Subtract1/1  "2^(d-NShifts)"
  Constant/1 -> LSR(N)/2(x_in)
  Subtract/1 -> Product2/1  "Delta_LUT"
  LUT_low/1 -> Relational Operator/1, Switch1/1, Subtract3/1, Switch/1, Subtract/1
  LUT_high/1 -> Relational Operator/2, Subtract/2
  Bit Slice1/1 -> Product1/2  "M"
  Bitwise Operator/1 -> LSL(N)/1(NShifts), LSR(N)/1(NShifts)  "NShifts"
  Bit Slice/1 -> Bitwise Operator/1
  addr_low/1 -> Bit Slice/1, Bit Slice1/1
  Relational Operator/1 -> Switch1/2
  Switch1/1 -> Unit Delay/1

== system FPGA_Open_Speech_Tools/Programmable Lookup Table dB/LogAddressing ==
  note: z-1 here
      |    	|
      |    	|
      |   	v
  note: If input > highest expected input,
  note: If input < floor threshold input,
      | use the output corresponding to
      | the floor threshold input.
  note: Note: simulation version of this block has no latency.
      | But, in VHDL the inputs are registered, delaying the signal by 1.
      | If testing a simulation, simply attach a unit delay block after the
      | addition and before the signal split.
  note: Have to change size to 40 because
      |  LZC made for 40 bit number
  note: EFFECTIVELY shift_left(x_in,NShifts)
  x_in : Inport
  Bit Concat : hdlsllib/Logic and Bit Operations/Bit Concat  numInputs=2
  Bit Slice : hdlsllib/Logic and Bit Operations/Bit Slice  lidx=N_bits-1  ridx=0
      settings: SourceProductBaseCode=SL
  Bit Slice1 : hdlsllib/Logic and Bit Operations/Bit Slice  lidx=F_bits-1+binaryOffset  ridx=F_bits-M_bits+binaryOffset
      settings: SourceProductBaseCode=SL
  Bitwise Operator1 : simulink/Logic and Bit Operations/Bitwise Operator  logicop=NOT  UseBitMask=off  BitMask=bin2dec('11011001')  BitMaskRealWorld=Stored Integer
  Constant6 : Constant  Value=0  OutDataTypeStr=fixdt(0,RAM_SIZE,0)  SampleTime=-1
  Data Type Conversion : DataTypeConversion  OutDataTypeStr=fixdt(0,40,F_bits+40-W_bits)
  Delay1 : Delay  DelayLength=1  InitialCondition=minVal
  Delay2 : Delay  DelayLength=1  InitialCondition=minVal
  LSL(N) : Subsystem
  MATLAB Function : MATLAB Function  TreatAsAtomicUnit=on
  Offset : Constant  Value=W_bits-1-F_bits-binaryOffset  OutDataTypeStr=fixdt(0,6,0)  SampleTime=-1
  Remove Sign : DataTypeConversion  OutDataTypeStr=fixdt(0,W_bits,F_bits)
  Subtract : Sum  Inputs=+-  OutDataTypeStr=Inherit: Same as first input
  Switch1 : Switch  Criteria=u2 ~= 0
  Threshold Check : simulink/Logic and Bit Operations/Compare To Constant  relop=>  const=2^N_bits -1  OutDataTypeStr=boolean
  addr_r : Outport  VectorParamsAs1DForOutWhenUnconnected=off
  wires:
  x_in/1 -> Remove Sign/1, Data Type Conversion/1
  Bit Slice1/1 -> Bit Concat/2  "M"
  Bitwise Operator1/1 -> Bit Concat/1  "addr(5 downto 2)"
  MATLAB Function/1(lzc_count) -> Subtract/1
  Bit Concat/1 -> Switch1/3
  Offset/1 -> Subtract/2
  Bit Slice/1 -> Bitwise Operator1/1, LSL(N)/1(NShifts)  "NShifts"
  Delay2/1 -> LSL(N)/2(x_in)
  LSL(N)/1(x_shifted) -> Bit Slice1/1
  Data Type Conversion/1 -> MATLAB Function/1(x)
  Constant6/1 -> Switch1/1
  Switch1/1 -> addr_r/1
  Threshold Check/1 -> Switch1/2
  Remove Sign/1 -> Delay2/1
  Subtract/1 -> Delay1/1
  Delay1/1 -> Threshold Check/1, Bit Slice/1

== system FPGA_Open_Speech_Tools/Programmable Upclocked FIR/Addr_Gen  ==
  note: Realign Delay here?
  Add : Sum  OutDataTypeStr=Inherit: Same as first input
  Compare To Zero : simulink/Logic and Bit Operations/Compare To Zero  relop===  OutDataTypeStr=boolean  ZeroCross=off
  Constant : Constant  OutDataTypeStr=fixdt(0, FIR_SIZE,0)  SampleTime=-1
  Counter 0 to |b_k|-1 : simulink/Sources/Counter Free-Running  NumBits=FIR_SIZE  tsamp=Ts/FIR_UPRATE
  Input_Addr_Counter : simulink/Sources/Counter Free-Running  NumBits=FIR_SIZE  tsamp=Ts
  Rate Transition : RateTransition  OutPortSampleTime=Ts/FIR_UPRATE
  Realignment_delay : Constant  Value=rotationDelay  OutDataTypeStr=fixdt(0, FIR_SIZE,0)  SampleTime=Ts/FIR_UPRATE
  Subtract : Sum  Inputs=+--  OutDataTypeStr=Inherit: Same as first input
  Input_Addr : Outport  VectorParamsAs1DForOutWhenUnconnected=off
  Data_History_Rd_addr : Outport  Port=2  VectorParamsAs1DForOutWhenUnconnected=off
  End_of_sample_calc : Outport  Port=3  VectorParamsAs1DForOutWhenUnconnected=off
  b_k_addr : Outport  Port=4  VectorParamsAs1DForOutWhenUnconnected=off
  wires:
  Counter 0 to |b_k|-1/1 -> Compare To Zero/1, b_k_addr/1, Subtract/2
  Subtract/1 -> Data_History_Rd_addr/1
  Input_Addr_Counter/1 -> Rate Transition/1
  Add/1 -> Input_Addr/1
  Constant/1 -> Add/2
  Realignment_delay/1 -> Subtract/3
  Compare To Zero/1 -> End_of_sample_calc/1
  Rate Transition/1 -> Subtract/1, Add/1

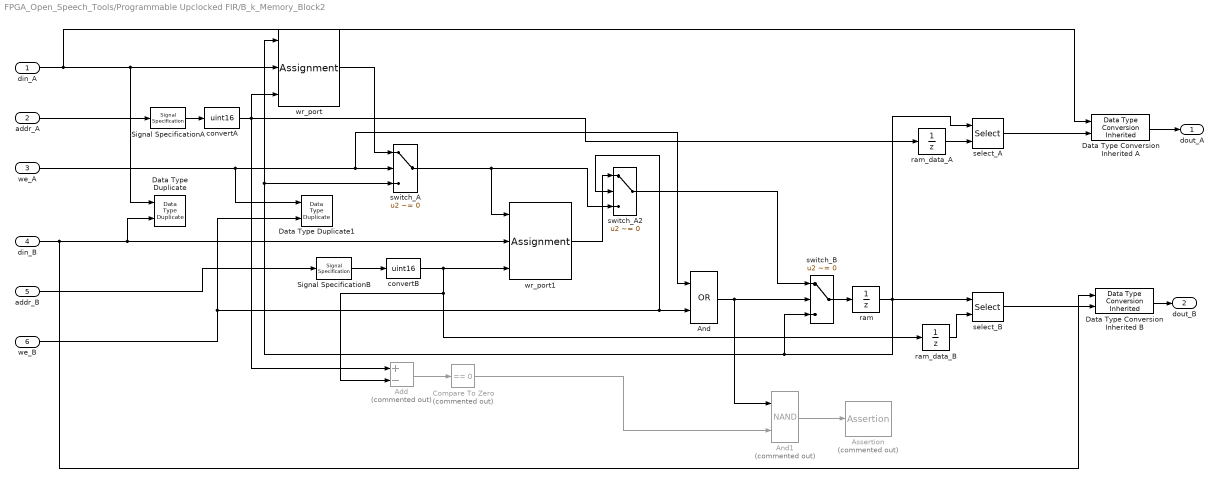
== system FPGA_Open_Speech_Tools/Programmable Upclocked FIR/B_k_Memory_Block2 ==
  din_A : Inport
  addr_A : Inport  Port=2
  we_A : Inport  Port=3  OutDataTypeStr=boolean
  din_B : Inport  Port=4
  addr_B : Inport  Port=5
  we_B : Inport  Port=6  OutDataTypeStr=boolean
  Add : Sum  Commented=on  Inputs=+-
  And : Logic  Operator=OR  AllPortsSameDT=off  OutDataTypeStr=boolean
  And1 : Logic  Commented=on  Operator=NAND  AllPortsSameDT=off  OutDataTypeStr=boolean
  Assertion : Assertion  Commented=on  StopWhenAssertionFail=off
  Compare To Zero : simulink/Logic and Bit Operations/Compare To Zero  Commented=on  relop===  OutDataTypeStr=boolean
  Data Type Conversion Inherited A : simulink/Signal Attributes/Data Type Conversion Inherited  ConvertRealWorld=Real World Value  DoSatur=off
      settings: SourceProductBaseCode=SL
  Data Type Conversion Inherited B : simulink/Signal Attributes/Data Type Conversion Inherited  ConvertRealWorld=Real World Value  DoSatur=off
      settings: SourceProductBaseCode=SL
  Data Type Duplicate : DataTypeDuplicate
  Data Type Duplicate1 : DataTypeDuplicate
  Signal SpecificationA : SignalSpecification  OutDataTypeStr=fixdt(0,ram_size,0)  Dimensions=1
  Signal SpecificationB : SignalSpecification  OutDataTypeStr=fixdt(0,ram_size,0)  Dimensions=1
  convertA : DataTypeConversion  OutDataTypeStr=uint16
  convertB : DataTypeConversion  OutDataTypeStr=uint16
  ram : UnitDelay  InitialCondition=B_k_init  SampleTime=-1  HasFrameUpgradeWarning=on
  ram_data_A : UnitDelay  SampleTime=-1  HasFrameUpgradeWarning=on
  ram_data_B : UnitDelay  SampleTime=-1  HasFrameUpgradeWarning=on
  select_A : Selector  IndexMode=Zero-based  InputPortWidth=2^ram_size  IndexOptions=Index vector (port)  Indices=[1 3]  OutputSizes=1
  select_B : Selector  IndexMode=Zero-based  InputPortWidth=2^ram_size  IndexOptions=Index vector (port)  Indices=[1 3]  OutputSizes=1
  switch_A : Switch  Criteria=u2 ~= 0
  switch_A2 : Switch  Criteria=u2 ~= 0
  switch_B : Switch  Criteria=u2 ~= 0
  wr_port : Assignment  IndexMode=Zero-based  IndexOptions=Index vector (port)  Indices=1  OutputSizes=[1 1]
  wr_port1 : Assignment  IndexMode=Zero-based  IndexOptions=Index vector (port)  Indices=1  OutputSizes=[1 1]
  dout_A : Outport  VectorParamsAs1DForOutWhenUnconnected=off
  dout_B : Outport  Port=2  VectorParamsAs1DForOutWhenUnconnected=off
  wires:
  switch_A2/1 -> switch_B/1
  And1/1 -> Assertion/1
  Signal SpecificationA/1 -> convertA/1
  Signal SpecificationB/1 -> convertB/1
  switch_B/1 -> ram/1
  convertA/1 -> ram_data_A/1, wr_port/3, Add/1
  ram/1 -> select_B/1, switch_B/3, switch_A/3, wr_port/1, select_A/1
  wr_port/1 -> switch_A/1
  And/1 -> And1/1, switch_B/2
  wr_port1/1 -> switch_A2/1
  Add/1 -> Compare To Zero/1
  Compare To Zero/1 -> And1/2
  we_B/1 -> switch_A2/2, And/2, Data Type Duplicate1/2
  switch_A/1 -> wr_port1/1, switch_A2/3
  addr_B/1 -> Signal SpecificationB/1
  ram_data_B/1 -> select_B/2
  we_A/1 -> Data Type Duplicate1/1, And/1, switch_A/2
  ram_data_A/1 -> select_A/2
  din_A/1 -> Data Type Duplicate/1, wr_port/2, Data Type Conversion Inherited A/1
  convertB/1 -> ram_data_B/1, Add/2, wr_port1/3
  din_B/1 -> wr_port1/2, Data Type Duplicate/2, Data Type Conversion Inherited B/1
  addr_A/1 -> Signal SpecificationA/1
  select_B/1 -> Data Type Conversion Inherited B/2
  Data Type Conversion Inherited B/1 -> dout_B/1
  select_A/1 -> Data Type Conversion Inherited A/2
  Data Type Conversion Inherited A/1 -> dout_A/1

== system FPGA_Open_Speech_Tools/Programmable Upclocked FIR/Multiply_And_Sum ==
  note: End_of_sample_calc triggers this subsystem to give the FIR output for this sample.
      | Also, it resets the sum memory back to 0.
  x[n-i] : Inport
  End_of_sample_calc : Inport  Port=2
  b_i : Inport  Port=3
  Bitwise Operator : simulink/Logic and Bit Operations/Bitwise Operator  logicop=NOT  UseBitMask=off  BitMask=bin2dec('11011001')  BitMaskRealWorld=Stored Integer
  Constant : Constant  Value=0  OutDataTypeStr=fixdt(1, W_bits, F_bits)  SampleTime=Ts/FIR_UPRATE
  Multiply-Add : hdlsllib/HDL Operations/Multiply-Add  Function=c+(a.*b)  datatype=Inherit: Same as first input  DoSatur=off  FMA=off
      settings: SourceProductBaseCode=SL
  Reset_Switch : Switch  Criteria=u2 ~= 0  ZeroCross=off
  Sum_memory : UnitDelay  SampleTime=-1  HasFrameUpgradeWarning=on
  convertB : DataTypeConversion  OutDataTypeStr=fixdt(1, W_bits, F_bits)
  Filtered_Output : Outport  VectorParamsAs1DForOutWhenUnconnected=off
  Output_Valid : Outport  Port=2  VectorParamsAs1DForOutWhenUnconnected=off
  wires:
  x[n-i]/1 -> Multiply-Add/1
  b_i/1 -> Multiply-Add/2
  Sum_memory/1 -> Reset_Switch/1, Filtered_Output/1
  Multiply-Add/1 -> convertB/1
  Reset_Switch/1 -> Multiply-Add/3
  Constant/1 -> Reset_Switch/3
  Bitwise Operator/1 -> Reset_Switch/2
  convertB/1 -> Sum_memory/1
  End_of_sample_calc/1 -> Output_Valid/1, Bitwise Operator/1

== system FPGA_Open_Speech_Tools/Static Upclocked FIR/Addr_Gen  ==
  note: Realign Delay here?
  Add : Sum  OutDataTypeStr=Inherit: Same as first input
  Compare To Zero : simulink/Logic and Bit Operations/Compare To Zero  relop===  OutDataTypeStr=boolean  ZeroCross=off
  Constant : Constant  OutDataTypeStr=fixdt(0, FIR_SIZE,0)  SampleTime=-1
  Counter 0 to |b_k|-1 : simulink/Sources/Counter Free-Running  NumBits=FIR_SIZE  tsamp=Ts/FIR_UPRATE
  Input_Addr_Counter : simulink/Sources/Counter Free-Running  NumBits=FIR_SIZE  tsamp=Ts
  Rate Transition : RateTransition  OutPortSampleTime=Ts/FIR_UPRATE
  Realignment_delay : Constant  Value=rotationDelay  OutDataTypeStr=fixdt(0, FIR_SIZE,0)  SampleTime=Ts/FIR_UPRATE
  Subtract : Sum  Inputs=+--  OutDataTypeStr=Inherit: Same as first input
  Input_Addr : Outport  VectorParamsAs1DForOutWhenUnconnected=off
  Data_History_Rd_addr : Outport  Port=2  VectorParamsAs1DForOutWhenUnconnected=off
  End_of_sample_calc : Outport  Port=3  VectorParamsAs1DForOutWhenUnconnected=off
  b_k_addr : Outport  Port=4  VectorParamsAs1DForOutWhenUnconnected=off
  wires:
  Counter 0 to |b_k|-1/1 -> Subtract/2, Compare To Zero/1, b_k_addr/1
  Subtract/1 -> Data_History_Rd_addr/1
  Input_Addr_Counter/1 -> Rate Transition/1
  Add/1 -> Input_Addr/1
  Constant/1 -> Add/2
  Realignment_delay/1 -> Subtract/3
  Compare To Zero/1 -> End_of_sample_calc/1
  Rate Transition/1 -> Subtract/1, Add/1
